simulink model "ftc_2AGENTS_sim"  (R2024a)
settings: Solver=VariableStepAuto  StartTime=0.0  StopTime=20  RelTol=1e-3
values from neighbouring files (symbols this model uses):
  csi_init = pos_init(:, 1) - pos_init(:, 2)    [ftc_2AGENTS.m]    (also in ftc_4AGENTS.m = d)
undefined symbols (not defined in the file or in its folder): param, pos_init
libraries: sim3dlib x3
settings Model: Creator=antor  LastModifiedBy=antor

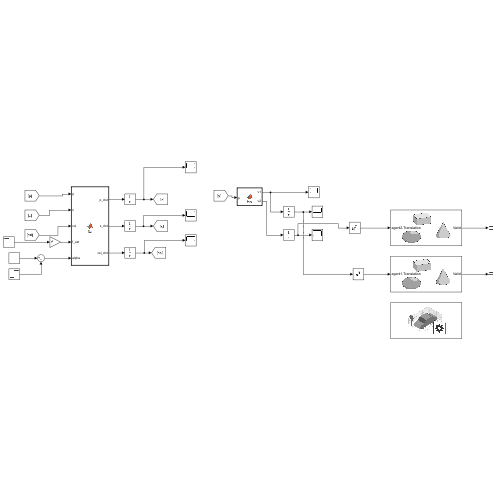
[thumbnail: Simulink's stored preview of the top-level diagram]
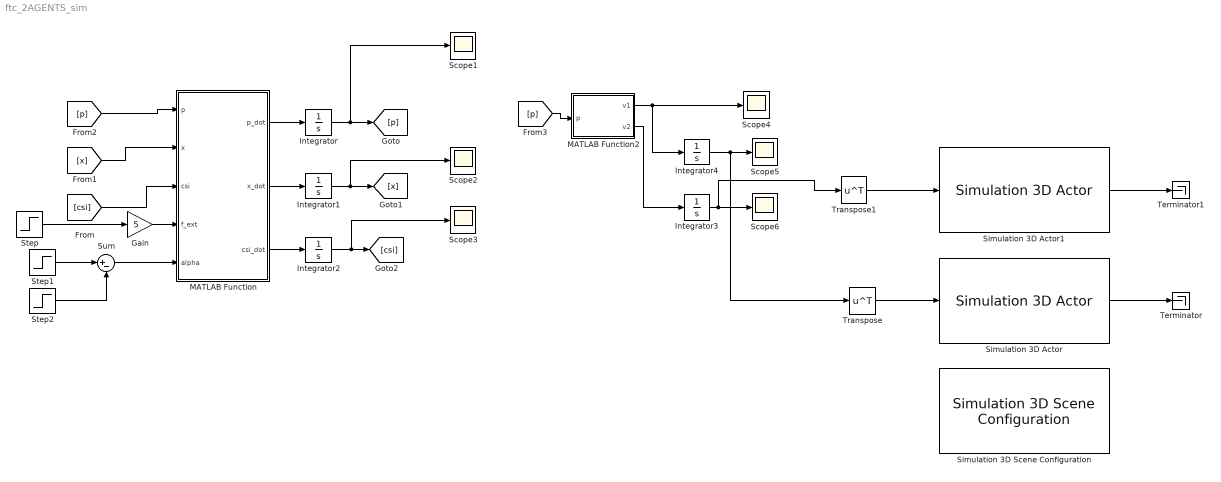
== system ftc_2AGENTS_sim ==
  Gain : Gain  Gain=5
  Integrator : Integrator  InitialCondition=zeros(3, param.N)
  Integrator1 : Integrator  InitialCondition=5*ones(1, param.N)
  Integrator2 : Integrator  InitialCondition=csi_init
  Integrator3 : Integrator  InitialCondition=pos_init(:, 2)
  Integrator4 : Integrator  InitialCondition=pos_init(:, 1)
  MATLAB Function : MATLAB Function  TreatAsAtomicUnit=on
  MATLAB Function2 : MATLAB Function  TreatAsAtomicUnit=on
  Scope{1..6} (6 alike) : Scope
  Simulation 3D Actor : sim3dlib/Simulation 3D Actor  Priority=1  ActorName=agent1  ParentName=Scene Origin  Operation=Create at setup  InitScriptText=|  SampleTime=-1  Translation=pos_init(:, 1).'  Rotation=single([0 0 0])  Scale=single([1 1 1])  InputsText=agent1.Translation  aMode=5  ActorTag=Sim3dActor1  ActorType=Sim3dActor  ID=1
      | Actor.createShape('sphere', [1 1 1]);
      | Actor.Scale = 0.1;
      | Actor.Color = [1 0 0];
  Simulation 3D Actor1 : sim3dlib/Simulation 3D Actor  Priority=1  ActorName=agent2  ParentName=Scene Origin  Operation=Create at setup  InitScriptText=|  SampleTime=-1  Translation=pos_init(:, 2).'  Rotation=single([0 0 0])  Scale=single([1 1 1])  InputsText=agent2.Translation  aMode=5  ActorTag=agent2  ActorType=Sim3dActor  ID=C
      | Actor.createShape('sphere', [1 1 1]);
      | Actor.Scale = 0.1;
      | Actor.Color = [0 1 0];
  Simulation 3D Scene Configuration : sim3dlib/Simulation 3D Scene Configuration  Priority=0  ProjectFormat=Default Scenes  SceneDesc=Empty scene  ProjectName=C:\Program Files\MATLAB\R2024a\toolbox\shared\sim3d_projects\automotive_project_windows\UE\WindowsNoEditor\VehicleSimulation.exe  ScenePath=/Game/Maps/HwStrght  EnableOpenDRIVE=off  vehTagList={'Custom';'Scene Origin';'agent1'}  vehTag=Scene Origin  FreeCameraInitialTranslation=[0, 0, 0]  FreeCameraDefaultInitialTranslation=[-6, 0, 2]  FreeCameraInitialRotation=[0, 0, 0]  FreeCameraDefaultInitialRotation=[0, -15, 0]  OpVisEn=off  Ts=.02  EnableWindow=on  EnableRemoteAccess=off  EnableWeather=off  SunAzimuth=90  SunAltitude=40.0  EnableGeospatialSun=off  Latitude=0  Longitude=0  Date=2023-01-01  Time=10:30:00  GeoTimeZone=-5.0  SunDaylightSaving=off  wind=1  clouds=10  EnableVolumetricClouds=off  CloudCoverage=0  CloudAltitude=6  fog=0  rain=0  RaindropsEffect=off  SnowDensity=0  EnableGeospatial=off  UseTrueOrigin=off  OriginHeight=200  OriginLatitude=40.744652  OriginLongitude=-73.988864  MapStyle=Aerial  AdditionalAssetIDs=[]  UseAdvancedSunSky=off  SolarTime=11  TimeZone=-5  Day=21  Month=9  Year=2022  UseDaylightSavingTime=on  DSTStartDay=10  DSTStartMonth=3  DSTEndDay=3  DSTEndMonth=11  DSTSwitchHour=2  sensorTag=MainCamera1  sensorId=1  sensorName=MainCamera1  mountLoc=Origin  offsetFlag=off  tmountOffset=[0, 0, 0]  rmountOffset=[0, 0, 0]  HorizontalResolution=1280  VerticalResolution=720  HorizontalFOV=60  mountPoint=[0 0 0]  mountOrientation=[0 0 0]  aMode=5  ID=1  GeoTrigger=Inactive
      settings: LibrarySourceBlock=sl3dlib/Simulation 3D/Environment/Simulation 3D Scene Configuration
  Step : Step  Time=3  Before=[1; 0; 0]  After=[0; 0; 0]  SampleTime=0
  Step1 : Step  Time=10  After=0.01  SampleTime=0
  Step2 : Step  Time=10.1  After=0.01  SampleTime=0
  Sum : Sum  Inputs=|+-
  Terminator : Terminator
  Terminator1 : Terminator
  Transpose : Math  Operator=transpose
  Transpose1 : Math  Operator=transpose
  wires:
  MATLAB Function/1(p_dot) -> Integrator/1
  MATLAB Function/2(x_dot) -> Integrator1/1
  MATLAB Function/3(csi_dot) -> Integrator2/1
  Integrator2/1 -> Scope3/1, [csi]
  Integrator1/1 -> Scope2/1, [x]
  Integrator/1 -> Scope1/1, [p]
  [csi] -> MATLAB Function/3(csi)
  [x] -> MATLAB Function/2(x)
  [p] -> MATLAB Function/1(p)
  Step/1 -> Gain/1
  [p] -> MATLAB Function2/1(p)
  MATLAB Function2/1(v1) -> Integrator4/1, Scope4/1
  Integrator4/1 -> Transpose/1, Scope5/1
  Gain/1 -> MATLAB Function/4(f_ext)
  Step1/1 -> Sum/1
  Step2/1 -> Sum/2
  Sum/1 -> MATLAB Function/5(alpha)
  Simulation 3D Actor/1 -> Terminator/1
  Transpose/1 -> Simulation 3D Actor/1
  Simulation 3D Actor1/1 -> Terminator1/1
  MATLAB Function2/2(v2) -> Integrator3/1
  Integrator3/1 -> Transpose1/1, Scope6/1
  Transpose1/1 -> Simulation 3D Actor1/1

== matlab function ftc_2AGENTS_sim/MATLAB Function ==
  data: p input; p_dot output; x input; csi input; f_ext input; alpha input; x_dot output; csi_dot output; param parameter
function [p_dot, x_dot, csi_dot] = ftc(p, x, csi, f_ext, alpha, param)
    N = param.N;
    N = 2;
    E = param.E;
    K = param.K;
    M = param.M;
    B = param.B;
    d = param.d;

    p_dot = zeros(3, N);
    x_dot = zeros(1, N);
    r = zeros(1, 3, N);
    h = zeros(1, 3, N);

    x = x';

    for i = 1:N
        r(:, :, i) = (B(:, :, i)*(M(:, :, i)\p(:, i))).'./repmat(x(:, i), 1, 3);
        h(:, :, i) = alpha*(K*(csi-d)*x(:, i)).';
    end

    csi_dot = zeros(3, 1);
    for i = 1:N
        p_dot(:, i) = - r(:, :, i).'*x(:, i) + E(i)*K*(csi-d);
        x_dot(:, i) = r(:, :, i)*(M(:, :, i)\p(:, i)) - h(:, :, i)*K*(csi-d);
        csi_dot = csi_dot - E(i)*(M(:, :, i)\p(:, i)) + h(:, :, i).'.*repmat(x(:, i), 3, 1);
    end
    p_dot(:, 1) = p_dot(:, 1) + f_ext;

end

== matlab function ftc_2AGENTS_sim/MATLAB Function2 ==
  data: v1 output; p input; param parameter; v2 output
function [v1, v2] = fcn(p, param)
    N = param.N;
    N = 2;
    M = param.M;

    v1 = M(:, :, 1)\p(:, 1);
    v2 = M(:, :, 2)\p(:, 2);
end
